simulink library "tqd"  (R2021b)
settings: Solver=VariableStepAuto  StartTime=0.0  StopTime=10.0  RelTol=1e-3
undefined symbols (not defined in the file or in its folder): ATQD_AccelLimitInRange_X_rpm, ATQD_AccelLimitInRange_Y_Nm, ATQD_AccelLimitOvrKi_X_Nm, ATQD_AccelLimitOvrKp_X_Nm, ATQD_BOSMapD_X_rpm, ATQD_BOSMapD_Y_pct, ATQD_BOSMapR_X_rpm, ATQD_BOSMapR_Y_pct, ATQD_HVBCurrSmooth_X_A, ATQD_LHMTqMapDLC_X_rpm, ATQD_LHMTqMapDLC_Y_pct, ATQD_LHMTqMapRLC_X_rpm, ATQD_LHMTqMapRLC_Y_pct, ATQD_NormalMapDLC_X_rpm, ATQD_NormalMapDLC_Y_pct, ATQD_NormalTqDecSR_X_rpm, ATQD_NormalTqDecSR_Y_Nm, ATQD_NormalTqIncSR_X_rpm, ATQD_NormalTqIncSR_Y_Nm, ATQD_OPDMapRLC_X_rpm, ATQD_OPDMapRLC_Y_pct, ATQD_RollRegTorReq_X_rpm, ATQD_RollRegTorReq_Y_enum, ATQD_VehSpdLimitInRange_X_rpm, ATQD_VehSpdLimitInRange_Y_Nm, ATQD_VehSpdLimitOvrKi_X_Nm, ATQD_VehSpdLimitOvrKp_X_Nm, EIGHT_INT, ENUM_BRAKEPEDAL_PRESSED, ENUM_BRAKEPEDAL_RELEASED, ENUM_COMBOKEY_DOWN, ENUM_COMBOKEY_M1, ENUM_COMBOKEY_M2, ENUM_COMBOKEY_NONE, ENUM_COMBOKEY_RKNEE, ENUM_COMBOKEY_STOPLV, ENUM_COMBOKEY_UP, ENUM_CP2VKNEEREQ_REQUEST, ENUM_CP2VNLVREQ_LEVEL1, ENUM_CP2VNLVREQ_LEVEL2, ENUM_CP2VNLVREQ_LOWER, ENUM_CP2VNLVREQ_STOPLV, ENUM_CP2VNLVREQ_UPPER, ENUM_CREEPIND_DISABLE, ENUM_CREEPIND_READY, ENUM_CREEPIND_RUNNING, ENUM_CREEPIND_WARNING, ENUM_DRIVELINERELEASE_RELEASE, ENUM_EBSTORQUERWQ_LIMIT, ENUM_EBSTORQUERWQ_TORQUE, ENUM_ECPVCUDRM_CONFORT, ENUM_ECPVCUDRM_ECO, ENUM_ECPVCUDRM_NORMAL, ENUM_ECPVCUDRM_NOTAVAILABLE, ENUM_EMTqModeDrvBrk_Accel, ENUM_EMTqModeDrvBrk_Brake, ENUM_EMTqModeDrvBrk_Coast, ENUM_ETC2ACTDRIVEDIR_BACKWARD, ENUM_ETC2ACTDRIVEDIR_FORWARD, ENUM_ETC2ACTDRIVEDIR_STILL ... (+341)
libraries: simulink x109, hcu_lib x67
(part 7 of 13)

== system tqd/TQD/Input_Convert/Function/Rolling Regen ==
  note: Torque Determination
  note: Enable Judgment
  BSCPIn_outputs : Inport
  BSignalConvert_outputs : Inport  Port=2
  VTQD_VCUMCUCtrlMdTQD_enum : Inport  Port=3
  AND : Logic  Inputs=8  AllPortsSameDT=off  OutDataTypeStr=boolean
  Bus Selector : BusSelector  OutputSignals=VTQD_EBSLostZeroReg_flg,VTQD_ActDriveMode_enum,VTQD_VCUVehSpd_kph
  Bus Selector1 : BusSelector  OutputSignals=VDHP_ActAPSPosn_pct,VINP_B2VAvaPlsChgCurr_A,VDMM_CAN1BUSOFF_flg,VINP_ECPVCURRegenSW_enum,VINP_EM1OvrCtrlMBrk_enum,VINP_MotorSpd_rpm,VINP_CANMsgValidECP3_flg
  Constant : Constant  Value=KTQD_RollRegAPSLimit_pct
  Constant1 : Constant  Value=KTQD_RollRegVehSpdLimit_kph
  Constant10 : Constant  Value=KTQD_RollingRegSW_enum_ovrdval
  Constant11 : Constant  Value=KTQD_RollingRegSW_enum_ovrdflg
  Constant12 : Constant  Value=KTQD_RollingRegSW_flg_ovrdflg
  Constant13 : Constant  Value=KTQD_RegenModeSW_flg
  Constant2 : Constant  Value=KTQD_RollRegBatAvalChgCurr_A
  Constant3 : Constant  Value=ENUM_MCUCTRLMODE_TORQUE
  Constant4 : Constant  Value=ZERO_FLOAT
  Constant5 : Constant  Value=KTQD_RollRegenIni_enum
  Constant6 : Constant  Value=KTQD_RollRegenThreshold_enum
  Constant7 : Constant  Value=ENUM_EBSTORQUERWQ_TORQUE
  Constant8 : Constant  Value=ZERO_INT
  Constant9 : Constant  Value=KTQD_RollingRegSW_flg_ovrdval
  Data Type Conversion : DataTypeConversion  OutDataTypeStr=single
  Data Type Conversion1 : DataTypeConversion  OutDataTypeStr=single
  Equal : RelationalOperator  Operator=~=  OutDataTypeStr=boolean  RndMeth=Simplest
  Gain1 : Gain  Gain=MINUSONE_FLOAT
  Gain2 : Gain  Gain=MINUSONE_FLOAT
  MTQD_RollRegTorReq_Z_Nm : Lookup_n-D  BreakpointsForDimension1=ATQD_RollRegTorReq_Y_enum  BreakpointsForDimension2=ATQD_RollRegTorReq_X_rpm  Table=MTQD_RollRegTorReq_Z_Nm  InternalRulePriority=Speed  RndMeth=Simplest  InputSameDT=on
      settings: InputPortMap=u0,u1
  MTQD_RollRegTorReq_Z_Nm1 : Lookup_n-D  BreakpointsForDimension1=ATQD_RollRegTorReq_Y_enum  BreakpointsForDimension2=ATQD_RollRegTorReq_X_rpm  Table=MTQD_RollRegTorReq_Z_Nm  InternalRulePriority=Speed  RndMeth=Simplest  InputSameDT=on
      settings: InputPortMap=u0,u1
  NOT : Logic  Operator=NOT  AllPortsSameDT=off  OutDataTypeStr=boolean
  NOT1 : Logic  Operator=NOT  AllPortsSameDT=off  OutDataTypeStr=boolean
  NOT2 : Logic  Operator=NOT  AllPortsSameDT=off  OutDataTypeStr=boolean
  OR : Logic  Operator=OR  AllPortsSameDT=off  OutDataTypeStr=boolean
  Relational Operator : RelationalOperator  Operator=<=  OutDataTypeStr=boolean  RndMeth=Simplest
  Relational Operator1 : RelationalOperator  OutDataTypeStr=boolean  RndMeth=Simplest
  Relational Operator2 : RelationalOperator  OutDataTypeStr=boolean  RndMeth=Simplest
  Relational Operator3 : RelationalOperator  Operator===  OutDataTypeStr=boolean  RndMeth=Simplest
  Relational Operator4 : RelationalOperator  Operator=>  OutDataTypeStr=boolean  RndMeth=Simplest
  Relational Operator5 : RelationalOperator  OutDataTypeStr=boolean  RndMeth=Simplest
  Switch{,2..4} (4 alike) : Switch  Criteria=u2 ~= 0
      settings: AttributesFormatString=%<Criteria>
  Switch1 : Switch  Criteria=u2 > Threshold
  VTQD_RollingRegenEnable_flg : Outport
  VTQD_RollRegTorReq_Nm : Outport  Port=2
  wires:
  [VTQD_RollingRegenEnable_flg] -> VTQD_RollingRegenEnable_flg/1
  BSCPIn_outputs/1 -> Bus Selector1/1
  Bus Selector/1 -> [VTQD_EBSLostZeroReg_flg]  "<VTQD_EBSLostZeroReg_flg>"
  BSignalConvert_outputs/1 -> Bus Selector/1
  [VINP_EM1OvrCtrlMBrk_enum] -> Equal/1
  Equal/1 -> AND/8
  Relational Operator5/1 -> Switch4/3
  Constant7/1 -> Equal/2
  Constant/1 -> Relational Operator/2
  Relational Operator2/1 -> AND/3
  Relational Operator1/1 -> AND/2
  [VDMM_CAN1BUSOFF_flg] -> NOT2/1
  [VINP_B2VAvaPlsChgCurr_A] -> Relational Operator2/1
  Relational Operator3/1 -> AND/4
  Relational Operator/1 -> AND/1
  [VTQD_VCUVehSpd_kph] -> Relational Operator1/1
  Constant8/1 -> Relational Operator5/2
  NOT1/1 -> AND/7
  Constant3/1 -> Relational Operator3/2
  Constant2/1 -> Relational Operator2/2
  [VINP_ECPVCURRegenSW_enum] -> Relational Operator5/1
  NOT2/1 -> AND/5
  Constant12/1 -> Switch4/2
  AND/1 -> [VTQD_RollingRegenEnable_flg]  "VTQD_RollingRegenEnable_flg"
  [VTQD_EBSLostZeroReg_flg] -> NOT1/1
  Switch4/1 -> AND/6
  Constant9/1 -> Switch4/1
  [VTQD_VCUMCUCtrlMdTQD_enum] -> Relational Operator3/1
  Constant1/1 -> Relational Operator1/2
  [VDHP_ActAPSPosn_pct] -> Relational Operator/1
  VTQD_VCUMCUCtrlMdTQD_enum/1 -> [VTQD_VCUMCUCtrlMdTQD_enum]
  MTQD_RollRegTorReq_Z_Nm1/1 -> Gain2/1
  Constant4/1 -> Switch/3
  Gain2/1 -> Switch1/3
  MTQD_RollRegTorReq_Z_Nm/1 -> Gain1/1
  Constant10/1 -> Switch3/1
  [VINP_MotorSpd_rpm] -> MTQD_RollRegTorReq_Z_Nm1/2
  Constant5/1 -> Data Type Conversion1/1
  Data Type Conversion1/1 -> MTQD_RollRegTorReq_Z_Nm/1
  [VINP_MotorSpd_rpm] -> MTQD_RollRegTorReq_Z_Nm/2
  Constant6/1 -> Relational Operator4/2
  Relational Operator4/1 -> OR/1
  [VINP_ECPVCURRegenSW_enum] -> Relational Operator4/1
  Switch3/1 -> Data Type Conversion/1
  OR/1 -> Switch1/2
  NOT/1 -> OR/2
  Gain1/1 -> Switch1/1
  Constant13/1 -> Switch2/2
  [VTQD_ActDriveMode_enum] -> Switch2/3
  Switch/1 -> [VTQD_RollRegTorReq_Nm]  "VTQD_RollRegTorReq_Nm"
  [VINP_CANMsgValidECP3_flg] -> NOT/1
  [VINP_ECPVCURRegenSW_enum] -> Switch2/1
  Switch1/1 -> Switch/1
  Constant11/1 -> Switch3/2
  [VTQD_RollingRegenEnable_flg] -> Switch/2
  Switch2/1 -> Switch3/3
  Data Type Conversion/1 -> MTQD_RollRegTorReq_Z_Nm1/1
  [VTQD_RollRegTorReq_Nm] -> VTQD_RollRegTorReq_Nm/1
  Bus Selector/2 -> [VTQD_ActDriveMode_enum]  "<VTQD_ActDriveMode_enum>"
  Bus Selector1/1 -> [VDHP_ActAPSPosn_pct]  "<VDHP_ActAPSPosn_pct>"
  Bus Selector1/2 -> [VINP_B2VAvaPlsChgCurr_A]  "<VINP_B2VAvaPlsChgCurr_A>"
  Bus Selector1/3 -> [VDMM_CAN1BUSOFF_flg]  "<VDMM_CAN1BUSOFF_flg>"
  Bus Selector1/4 -> [VINP_ECPVCURRegenSW_enum]  "<VINP_ECPVCURRegenSW_enum>"
  Bus Selector1/5 -> [VINP_EM1OvrCtrlMBrk_enum]  "<VINP_EM1OvrCtrlMBrk_enum>"
  Bus Selector1/6 -> [VINP_MotorSpd_rpm]  "<VINP_MotorSpd_rpm>"
  Bus Selector1/7 -> [VINP_CANMsgValidECP3_flg]  "<VINP_CANMsgValidECP3_flg>"
  Bus Selector/3 -> [VTQD_VCUVehSpd_kph]  "<VTQD_VCUVehSpd_kph>"

== system tqd/TQD/Input_Convert/Function/Shift Modul ==
  note: Actual Gear Position State Machine
  note: Shift Gear Command Judgment
  BSCPIn_outputs : Inport
  BSignalConvert_outputs : Inport  Port=2
  Bus Selector : BusSelector  OutputSignals=VTQD_DrivePositionOn_flg,VTQD_NeutralPositionOn_flg,VTQD_ReversePositionOn_flg,VTQD_BrkSWOn_flg,VTQD_EVDriveReady_flg,VTQD_IGNActive_flg,VTQD_EVCU1VehActDrvDir_enum,VTQD_GearFlashInd_flg,VTQD_DMSLossLimitGear_flg,VTQD_VCUVehSpd_kph
  Bus Selector1 : BusSelector  OutputSignals=task_time_s,VINP_MotorSpd_rpm,VDMM_DTCDMSRCIncorrect_flg,VINP_ParkBrakeSW_flg
  Constant : Constant  Value=ENUM_GEARSHIFTPOSN_R
  Constant1 : Constant  Value=ENUM_GEARSHIFTPOSN_INVALID
  Constant{10..14} (5 alike) : Constant  Value=FALSE
  Constant2 : Constant  Value=ENUM_GEARSHIFTPOSN_N
  Constant4 : Constant  Value=ENUM_GEARSHIFTPOSN_D
  Delay : Delay  DelayLength=1  InitialConditionSource=Input port
      settings: AttributesFormatString=%<InitialConditionSource>  InputPortMap=u0,p4
  Determine_Actual_Gear_Position : Stateflow chart  TreatAsAtomicUnit=on
  Logical Operator : Logic  Operator=OR  Inputs=3  AllPortsSameDT=off  OutDataTypeStr=boolean
  Switch1 : Switch  Criteria=u2 ~= 0
      settings: AttributesFormatString=%<Criteria>
  Switch3 : Switch  Criteria=u2 ~= 0
      settings: AttributesFormatString=%<Criteria>
  Switch4 : Switch  Criteria=u2 ~= 0
      settings: AttributesFormatString=%<Criteria>
  VTQD_GearActualPosn_enum : Outport
  VTQD_ParkingPawlPwrOn_flg : Outport  Port=2
  VTQD_ParkingPawlEnable_flg : Outport  Port=3
  wires:
  BSignalConvert_outputs/1 -> Bus Selector/1
  Delay/1 -> Switch3/3
  Constant/1 -> Switch3/1
  Constant2/1 -> Switch4/1
  Switch4/1 -> Delay/1, [VTQD_GearShiftPosn_enum]  "VTQD_GearShiftPosn_enum"
  Switch3/1 -> Switch1/3
  Logical Operator/1 -> [VTQD_RNDTrig_flg]  "VTQD_RNDTrig_flg"
  Constant4/1 -> Switch1/1
  Constant1/1 -> Delay/2
  Switch1/1 -> Switch4/3
  Bus Selector/1 -> [VTQD_DrivePositionOn_flg]  "<VTQD_DrivePositionOn_flg>"
  Bus Selector/2 -> [VTQD_NeutralPositionOn_flg]  "<VTQD_NeutralPositionOn_flg>"
  Bus Selector/3 -> [VTQD_ReversePositionOn_flg]  "<VTQD_ReversePositionOn_flg>"
  [VTQD_NeutralPositionOn_flg] -> Switch4/2
  [VTQD_DrivePositionOn_flg] -> Switch1/2
  [VTQD_ReversePositionOn_flg] -> Switch3/2
  [VTQD_ReversePositionOn_flg] -> Logical Operator/3
  [VTQD_DrivePositionOn_flg] -> Logical Operator/2
  [VTQD_NeutralPositionOn_flg] -> Logical Operator/1
  Determine_Actual_Gear_Position/3(VTQD_ParkingPawlEnable_flg) -> [VTQD_ParkingPawlEnable_flg]
  Determine_Actual_Gear_Position/2(VTQD_ParkingPawlPwrOn_flg) -> [VTQD_ParkingPawlPwrOn_flg]
  [VDMM_DTCDMSRCIncorrect_flg] -> Determine_Actual_Gear_Position/17(VDMM_DTCDMSRCIncorrect_flg)
  [VINP_ParkBrakeSW_flg] -> Determine_Actual_Gear_Position/18(VINP_ParkBrakeSW_flg)
  [VTQD_GearFlashInd_flg] -> Determine_Actual_Gear_Position/14(VSCP_GearFlashInd_flg)
  [VTQD_EVCU1VehActDrvDir_enum] -> Determine_Actual_Gear_Position/13(VSCP_EVCU1VehActDrvDir_enum)
  [VTQD_EVDriveReady_flg] -> Determine_Actual_Gear_Position/6(VFUN_EVDriveReady_flg)
  [VTQD_tasktime_s] -> Determine_Actual_Gear_Position/5(task_time_s)
  [VTQD_BrkSWOn_flg] -> Determine_Actual_Gear_Position/4(VINP_BrkSwOn_flg)
  [VINP_MotorSpd_rpm] -> Determine_Actual_Gear_Position/16(VINP_TMSpd_rpm)
  [VTQD_DMSLossLimitGear_flg] -> Determine_Actual_Gear_Position/15(VTQD_DMSLossLimitGear_flg)
  [VTQD_GearShiftPosn_enum] -> Determine_Actual_Gear_Position/1(VTQD_GearShiftPosn_enum)
  [VTQD_VCUVehSpd_kph] -> Determine_Actual_Gear_Position/2(VINP_VehSpd_kph)
  [VTQD_RNDTrig_flg] -> Determine_Actual_Gear_Position/8(VTQD_RNDTrig_flg)
  Constant12/1 -> Determine_Actual_Gear_Position/10(VTQD_ADASModeDisact_flg)  "VTQD_ADASModeDisact_flg"
  [VTQD_IGNActive_flg] -> Determine_Actual_Gear_Position/7(VPSA_IGNActive_flg)
  Determine_Actual_Gear_Position/1(VTQD_GearActualPosn_enum) -> [VTQD_GearActualPosn_enum]
  BSCPIn_outputs/1 -> Bus Selector1/1
  Constant10/1 -> Determine_Actual_Gear_Position/3(VINP_ParkingPawlLock_flg)  "VINP_ParkingPawlLock_flg"
  Bus Selector/4 -> [VTQD_BrkSWOn_flg]  "<VTQD_BrkSWOn_flg>"
  Bus Selector/5 -> [VTQD_EVDriveReady_flg]  "<VTQD_EVDriveReady_flg>"
  Bus Selector/6 -> [VTQD_IGNActive_flg]  "<VTQD_IGNActive_flg>"
  Constant11/1 -> Determine_Actual_Gear_Position/9(VTQD_AutoPark_flg)  "VTQD_AutoPark_flg"
  Constant13/1 -> Determine_Actual_Gear_Position/11(VTQD_ExtShiftAvail_flg)  "VTQD_ExtShiftAvail_flg"
  Constant14/1 -> Determine_Actual_Gear_Position/12(VINP_ADASShftPosnReqA_flg)  "VINP_ADASShftPosnReqA_flg"
  Bus Selector/7 -> [VTQD_EVCU1VehActDrvDir_enum]  "<VTQD_EVCU1VehActDrvDir_enum>"
  Bus Selector/8 -> [VTQD_GearFlashInd_flg]  "<VTQD_GearFlashInd_flg>"
  Bus Selector/9 -> [VTQD_DMSLossLimitGear_flg]  "<VTQD_DMSLossLimitGear_flg>"
  [VTQD_GearActualPosn_enum] -> VTQD_GearActualPosn_enum/1
  [VTQD_ParkingPawlPwrOn_flg] -> VTQD_ParkingPawlPwrOn_flg/1
  [VTQD_ParkingPawlEnable_flg] -> VTQD_ParkingPawlEnable_flg/1
  Bus Selector1/1 -> [VTQD_tasktime_s]  "<task_time_s>"
  Bus Selector1/2 -> [VINP_MotorSpd_rpm]  "<VINP_MotorSpd_rpm>"
  Bus Selector1/3 -> [VDMM_DTCDMSRCIncorrect_flg]  "<VDMM_DTCDMSRCIncorrect_flg>"
  Bus Selector1/4 -> [VINP_ParkBrakeSW_flg]  "<VINP_ParkBrakeSW_flg>"
  Bus Selector/10 -> [VTQD_VCUVehSpd_kph]  "<VTQD_VCUVehSpd_kph>"

== system tqd/TQD/Input_Convert/Function/Speed Limiter ==
  note: Limit Speed Determination
  note: Torque Calculation
  note: Enable Judgment
  note: Signal Convert
  BSCPIn_outputs : Inport
  BSignalConvert_outputs : Inport  Port=2
  VTQD_GearActualPosn_enum : Inport  Port=3
  VTQD_PedalMapTq_Nm : Inport  Port=4
  AND : Logic  Inputs=6  AllPortsSameDT=off  OutDataTypeStr=boolean
  Add2 : Sum  Inputs=+-
  Add4 : Sum
  Bus Selector : BusSelector  OutputSignals=VTQD_PTAvailMotTq_Nm,VTQD_VCUVehSpd_kph
  Bus Selector1 : BusSelector  OutputSignals=task_time_s,VINP_ECPVCUSpdLim_kph,VINP_CANMsgValidECP2_flg,VINP_FASpeedValid_flg,VINP_MotorSpdValid_flg,VINP_ECPVCUSpdLimSw_flg,VINP_MotorSpd_rpm
  Constant : Constant  Value=SINGLEMAXCNT  OutDataTypeStr=single
  Constant1 : Constant  Value=KTQD_VehSpdLimitTG_kph
  Constant10 : Constant  Value=KTQD_VehSpdLimitSW_flg_ovrdval
  Constant11 : Constant  Value=KTQD_VehSpdOvrLimitRefreTime_s
  Constant12 : Constant  Value=KTQD_VehSpdLimitOvrRangeDis_kph
  Constant14 : Constant  Value=KTQD_VehSpdLimitTorLowerLim_Nm
  Constant15 : Constant  Value=KTQD_MCUMaxRefTorq_Nm
  Constant16 : Constant  Value=KTQD_VehSpdLimitSW_flg_ovrdflg
  Constant2 : Constant  Value=KTQD_VehSpdPhyShrehold_kph
  Constant3 : Constant  Value=KTQD_VehSpdLimitExtre_kph
  Constant4 : Constant  Value=KTQD_ECPSetValErr1_kph
  Constant5 : Constant  Value=KTQD_VehSpdLimitTG_kph
  Constant6 : Constant  Value=KTQD_ECPSetValNoReq_kph
  Constant7 : Constant  Value=ENUM_GEARACTUALPOSN_D
  Constant8 : Constant  Value=KTQD_VehSpdLimitInRangeDis_kph
  Constant9 : Constant  Value=KTQD_VehSpdOvrLimitRefreTime_s
  Counter : hcu_lib/Basic_Blocks/Counter
  Data Type Conversion : DataTypeConversion  OutDataTypeStr=single
  Detect Increase1 : simulink/Logic and Bit Operations/Detect Increase  vinit=boolean(0)  OutDataTypeStr=boolean
  Detect Increase3 : simulink/Logic and Bit Operations/Detect Increase  vinit=boolean(0)  OutDataTypeStr=boolean
  Equal : RelationalOperator  Operator===  OutDataTypeStr=boolean  RndMeth=Simplest
  Limit Torque Calculation : Subsystem  TreatAsAtomicUnit=on
  Limit2 : hcu_lib/Basic_Blocks/Limit
  MTQD_VehSpdLimitInRange_Z_Gain : Lookup_n-D  BreakpointsForDimension1=ATQD_VehSpdLimitInRange_Y_Nm  BreakpointsForDimension2=ATQD_VehSpdLimitInRange_X_rpm  Table=MTQD_VehSpdLimitInRange_Z_Gain  InternalRulePriority=Speed  RndMeth=Simplest  InputSameDT=on
      settings: InputPortMap=u0,u1
  Min : MinMax  Inputs=2
  NOT : Logic  Operator=NOT  AllPortsSameDT=off  OutDataTypeStr=boolean
  NOT1 : Logic  Operator=NOT  AllPortsSameDT=off  OutDataTypeStr=boolean
  NOT2 : Logic  Operator=NOT  AllPortsSameDT=off  OutDataTypeStr=boolean
  OR : Logic  Operator=OR  AllPortsSameDT=off  OutDataTypeStr=boolean
  Product : Product
  Product1 : Product
  Relational Operator{1..4} (4 alike) : RelationalOperator  OutDataTypeStr=boolean  RndMeth=Simplest
  Relational Operator11 : RelationalOperator  Operator=<  OutDataTypeStr=boolean  RndMeth=Simplest
  Relational Operator9 : RelationalOperator  Operator=<=  OutDataTypeStr=boolean  RndMeth=Simplest
  SR_Latch : hcu_lib/Basic_Blocks/SR_Latch
  Saturation : Saturate  UpperLimit=KTQD_MCUMaxRefTorq_Nm  LowerLimit=ZERO_FLOAT
      settings: AttributesFormatString=|
      | UpperLimit:%<UpperLimit>
      | LowerLimit:%<LowerLimit>
  Saturation1 : Saturate  UpperLimit=KTQD_EMSpdAcclLimitEnHi_rpm  LowerLimit=ZERO_FLOAT
      settings: AttributesFormatString=|
      | UpperLimit:%<UpperLimit>
      | LowerLimit:%<LowerLimit>
  Switch{1..3,5,10,12..13} (7 alike) : Switch  Criteria=u2 ~= 0
      settings: AttributesFormatString=%<Criteria>
  Unit Delay : UnitDelay  InitialCondition=boolean(0)  SampleTime=-1  HasFrameUpgradeWarning=on
      settings: AttributesFormatString=%<InitialCondition>
  Unit Delay1 : UnitDelay  InitialCondition=single(0)  SampleTime=-1  HasFrameUpgradeWarning=on
      settings: AttributesFormatString=%<InitialCondition>
  Unit Delay12 : UnitDelay  InitialCondition=THOUSAND  SampleTime=-1  HasFrameUpgradeWarning=on
      settings: AttributesFormatString=%<InitialCondition>
  VTQD_VehSpdLimitEnable_flg : Outport
  VTQD_VehSpdLimitTG_kph : Outport  Port=2
  VTQD_VehSpdTorLimit_Nm : Outport  Port=3
  wires:
  [VTQD_VehSpdLimitEnable_flg] -> VTQD_VehSpdLimitEnable_flg/1
  BSCPIn_outputs/1 -> Bus Selector1/1
  Bus Selector/1 -> [VTQD_PTAvailMotTq_Nm]  "<VTQD_PTAvailMotTq_Nm>"
  BSignalConvert_outputs/1 -> Bus Selector/1
  Constant2/1 -> Switch2/3
  [VTQD_VehSpdLimitEnable_flg] -> Switch2/2
  Switch2/1 -> [VTQD_VehSpdLimitRef_kph]  "VTQD_VehSpdLimitRef_kph"
  [VTQD_VehSpdLimitTG_kph] -> Switch2/1
  [VTQD_VehSpdLimitRef_kph] -> Add2/1
  Add2/1 -> Relational Operator1/2
  Add4/1 -> Relational Operator3/2
  Relational Operator1/1 -> [VTQD_VehSpdInLimit_flg]  "VTQD_VehSpdInLimit_flg"
  [VTQD_VCUVehSpd_kph] -> Relational Operator3/1
  Constant8/1 -> Add2/2
  [VTQD_VCUVehSpd_kph] -> Relational Operator1/1
  [VTQD_VehSpdLimitRef_kph] -> Add4/1
  Relational Operator4/1 -> [VTQD_VehSpdOvrRef_flg]  "VTQD_VehSpdOvrRef_flg"
  [VTQD_VehSpdLimitRef_kph] -> Relational Operator4/2
  Constant12/1 -> Add4/2
  [VTQD_VCUVehSpd_kph] -> Relational Operator4/1
  Relational Operator3/1 -> [VTQD_VehSpdOvrLimit_flg]  "VTQD_VehSpdOvrLimit_flg"
  [task_time_s] -> Product/2
  Product/1 -> Relational Operator2/1
  [VTQD_VehSpdOvrLimit_flg] -> NOT1/1, Counter/1
  Constant/1 -> Counter/3
  Unit Delay/1 -> OR/2
  Counter/1 -> Product/1
  OR/1 -> Counter/2
  Constant9/1 -> Relational Operator2/2
  Relational Operator2/1 -> [VTQD_VehSpdContiOvrLimit_flg], Unit Delay/1  "VTQD_VehSpdContiOvrLimit_flg"
  NOT1/1 -> OR/1
  [VINP_FASpeedValid_flg] -> AND/3
  AND/1 -> [VTQD_VehSpdLimitEnable_flg]  "VTQD_VehSpdLimitEnable_flg"
  [VINP_MotorSpdValid_flg] -> AND/5
  Constant4/1 -> Relational Operator11/2
  Switch5/1 -> AND/6
  Constant7/1 -> Equal/2
  [VINP_ECPVCUSpdLim_kph] -> Relational Operator11/1
  Equal/1 -> AND/1
  Relational Operator11/1 -> AND/4
  [VINP_CANMsgValidECP2_flg] -> AND/2
  [VTQD_GearActualPosn_enum] -> Equal/1
  Constant16/1 -> Switch5/2
  Constant10/1 -> Switch5/1
  [VINP_ECPVCUSpdLimSw_flg] -> Switch5/3
  [VINP_MotorSpd_rpm] -> Saturation1/1
  SR_Latch/1 -> NOT2/1
  Data Type Conversion/1 -> Switch12/1
  NOT/1 -> SR_Latch/2
  Switch13/1 -> Switch10/3
  Switch12/1 -> Limit2/1
  Constant15/1 -> Limit2/2
  [VTQD_VCUVehSpd_kph] -> Limit Torque Calculation/2(VDIP_VCUVehSpd_kph)
  [VTQD_VehSpdContiOvrLimit_flg] -> Limit Torque Calculation/Trigger
  Limit2/1 -> [VTQD_VehSpdTorLimit_Nm]  "VTQD_VehSpdTorLimit_Nm"
  Detect Increase1/1 -> SR_Latch/1
  Saturation/1 -> MTQD_VehSpdLimitInRange_Z_Gain/1
  [VTQD_PedalMapTq_Nm] -> Product1/2
  Saturation1/1 -> MTQD_VehSpdLimitInRange_Z_Gain/2
  MTQD_VehSpdLimitInRange_Z_Gain/1 -> Product1/1
  [VTQD_VehSpdInLimit_flg] -> Detect Increase1/1
  [VTQD_VehSpdContiOvrLimit_flg] -> Switch12/2
  [VTQD_PTAvailMotTq_Nm] -> Switch13/1
  Detect Increase3/1 -> Switch10/2
  Switch10/1 -> Switch12/3
  Unit Delay12/1 -> Switch13/3
  [VTQD_VehSpdInLimit_flg] -> Detect Increase3/1
  [VTQD_VehSpdOvrRef_flg] -> NOT/1
  [VTQD_VehSpdTorLimit_Nm] -> Unit Delay12/1
  Limit Torque Calculation/1(Result) -> Data Type Conversion/1
  [VTQD_VehSpdTorLimit_Nm] -> Unit Delay1/1
  [VTQD_PedalMapTq_Nm] -> Saturation/1
  Product1/1 -> Switch10/1
  Constant11/1 -> Limit Torque Calculation/3(PIControl_Task_time)
  Unit Delay1/1 -> Limit Torque Calculation/4(VTQD_VehSpdTorLimitLast_Nm)
  Constant14/1 -> Limit2/3
  [VTQD_VehSpdLimitRef_kph] -> Limit Torque Calculation/1(Refference)
  NOT2/1 -> Switch13/2
  Min/1 -> Switch3/1
  [VTQD_VehSpdLimitEnable_flg] -> Switch3/2
  Constant3/1 -> Switch3/3
  Switch1/1 -> Min/2
  Constant5/1 -> Switch1/1
  [VINP_ECPVCUSpdLim_kph] -> Relational Operator9/1
  Constant1/1 -> Min/1
  Relational Operator9/1 -> Switch1/2
  [VINP_ECPVCUSpdLim_kph] -> Switch1/3
  Constant6/1 -> Relational Operator9/2
  Switch3/1 -> [VTQD_VehSpdLimitTG_kph]  "VTQD_VehSpdLimitTG_kph"
  VTQD_GearActualPosn_enum/1 -> [VTQD_GearActualPosn_enum]
  VTQD_PedalMapTq_Nm/1 -> [VTQD_PedalMapTq_Nm]
  [VTQD_VehSpdLimitTG_kph] -> VTQD_VehSpdLimitTG_kph/1
  [VTQD_VehSpdTorLimit_Nm] -> VTQD_VehSpdTorLimit_Nm/1
  Bus Selector/2 -> [VTQD_VCUVehSpd_kph]  "<VTQD_VCUVehSpd_kph>"
  Bus Selector1/1 -> [task_time_s]  "<task_time_s>"
  Bus Selector1/2 -> [VINP_ECPVCUSpdLim_kph]  "<VINP_ECPVCUSpdLim_kph>"
  Bus Selector1/3 -> [VINP_CANMsgValidECP2_flg]  "<VINP_CANMsgValidECP2_flg>"
  Bus Selector1/4 -> [VINP_FASpeedValid_flg]  "<VINP_FASpeedValid_flg>"
  Bus Selector1/5 -> [VINP_MotorSpdValid_flg]  "<VINP_MotorSpdValid_flg>"
  Bus Selector1/6 -> [VINP_ECPVCUSpdLimSw_flg]  "<VINP_ECPVCUSpdLimSw_flg>"
  Bus Selector1/7 -> [VINP_MotorSpd_rpm]  "<VINP_MotorSpd_rpm>"

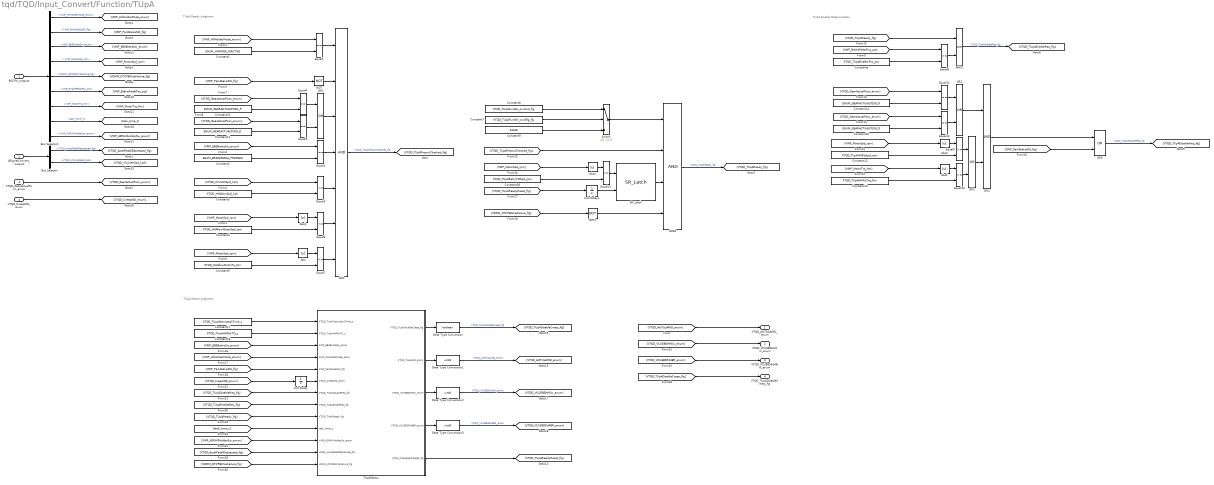
== system tqd/TQD/Input_Convert/Function/TUpA ==
  note: TUpA Status Judgment
  note: TUpA Ready Judgment
  note: TUpA Enable Determination
  BSCPIn_outputs : Inport
  BSignalConvert_outputs : Inport  Port=2
  VTQD_GearActualPosn_enum : Inport  Port=3
  VTQD_CreepIND_enum : Inport  Port=4
  AND : Logic  Inputs=7  AllPortsSameDT=off  OutDataTypeStr=boolean
  AND1 : Logic  AllPortsSameDT=off  OutDataTypeStr=boolean
  AND2 : Logic  Inputs=4  AllPortsSameDT=off  OutDataTypeStr=boolean
  Abs{,1..4} (5 alike) : Abs
  Bus Selector : BusSelector  OutputSignals=VTQD_AccelPedalDepressed_flg,VTQD_VCUVehSpd_kph
  Bus Selector1 : BusSelector  OutputSignals=VINP_HillHolderMode_enum,VINP_ParkBrakeSW_flg,VINP_EBSBrakeSw_enum,VINP_MotorSpd_rpm,VDMM_DTCPBWireFailure_flg,VINP_BrakePedalPos_pct,VINP_MotorTrq_Nm,task_time_s,VINP_ASRHillHolderSw_enum
  Constant1 : Constant  Value=ENUM_HHMODE_INACTIVE
  Constant10 : Constant  Value=ENUM_GEARACTUALPOSN_R
  Constant11 : Constant  Value=ENUM_GEARACTUALPOSN_D
  Constant12 : Constant  Value=KTQD_TUpAHHRlsSpd_rpm
  Constant13 : Constant  Value=KTQD_TUpAHHRlsTrq_Nm
  Constant14 : Constant  Value=ENUM_GEARACTUALPOSN_R
  Constant15 : Constant  Value=ENUM_GEARACTUALPOSN_D
  Constant16 : Constant  Value=KTQD_TUpAHHFbkTO_s
  Constant17 : Constant  Value=KTQD_TUpAWarnLatchTime_s
  Constant18 : Constant  Value=KTQD_TUpARetryTMSpd_rpm
  Constant2 : Constant  Value=ENUM_BRAKEPEDAL_PRESSED
  Constant3 : Constant  Value=KTQD_HHAllowSpd_kph
  Constant4 : Constant  Value=KTQD_HHAllowMotorSpd_rpm
  Constant5 : Constant  Value=KTQD_HHAllowMotorTq_Nm
  Constant6 : Constant  Value=KTQD_TUpAEnaBrkPos_pct
  Constant7 : Constant  Value=KTQD_TUpAFuncEn_ovrdflg_flg
  Constant8 : Constant  Value=KTQD_TUpAFuncEn_ovrdval_flg
  Constant9 : Constant  Value=FALSE
  Data Type Conversion : DataTypeConversion  OutDataTypeStr=boolean
  Data Type Conversion1 : DataTypeConversion  OutDataTypeStr=uint8
  Data Type Conversion2 : DataTypeConversion  OutDataTypeStr=uint8
  Data Type Conversion3 : DataTypeConversion  OutDataTypeStr=uint8
  Equal{1..2,4..5,11..12} (6 alike) : RelationalOperator  Operator===  OutDataTypeStr=boolean  RndMeth=Simplest
  Equal{8..10,13} (4 alike) : RelationalOperator  OutDataTypeStr=boolean  RndMeth=Simplest
  Equal3 : RelationalOperator  Operator=<=  OutDataTypeStr=boolean  RndMeth=Simplest
  Equal6 : RelationalOperator  Operator=<=  OutDataTypeStr=boolean  RndMeth=Simplest
  Equal7 : RelationalOperator  Operator=<=  OutDataTypeStr=boolean  RndMeth=Simplest
  NOT : Logic  Operator=NOT  AllPortsSameDT=off  OutDataTypeStr=boolean
  NOT1 : Logic  Operator=NOT  AllPortsSameDT=off  OutDataTypeStr=boolean
  OR{1..3,5} (4 alike) : Logic  Operator=OR  AllPortsSameDT=off  OutDataTypeStr=boolean
  OR4 : Logic  AllPortsSameDT=off  OutDataTypeStr=boolean
  SR_Latch : hcu_lib/Basic_Blocks/SR_Latch
      settings: SourceProductName=HCU Relative Block Library
  Switch : Switch  Criteria=u2 ~= 0
      settings: AttributesFormatString=%<Criteria>
  TUpAStatus : Stateflow chart  AncestorBlock=tqd_T1_A08133TT4/TQD/TorqueDemand/TorqueModule/TUpA/TUpAStatus  TreatAsAtomicUnit=on
  Unit Delay : UnitDelay  InitialCondition=uint8(0)  SampleTime=-1  HasFrameUpgradeWarning=on
      settings: AttributesFormatString=%<InitialCondition>
  Unit Delay1 : UnitDelay  InitialCondition=boolean(0)  SampleTime=-1  HasFrameUpgradeWarning=on
      settings: AttributesFormatString=%<InitialCondition>
  VTQD_ActTUpAIND_enum : Outport
  VTQD_VCUEBSHHSw_enum : Outport  Port=2
  VTQD_VCUEBSRd4BR_enum : Outport  Port=3
  VTQD_TUpADisableCreep_flg : Outport  Port=4
  wires:
  [VTQD_ActTUpAIND_enum] -> VTQD_ActTUpAIND_enum/1
  BSCPIn_outputs/1 -> Bus Selector1/1
  Bus Selector/1 -> [VTQD_AccelPedalDepressed_flg]  "<VTQD_AccelPedalDepressed_flg>"
  BSignalConvert_outputs/1 -> Bus Selector/1
  [VTQD_TUpAPreconChecked_flg] -> AND2/2
  Switch/1 -> AND2/1
  Constant2/1 -> Equal2/2
  Equal6/1 -> AND/6
  AND/1 -> [VTQD_TUpAPreconChecked_flg]  "VTQD_TUpAPreconChecked_flg"
  [VINP_EBSBrakeSw_enum] -> Equal2/1
  [VINP_ParkBrakeSW_flg] -> NOT/1
  [VTQD_VCUVehSpd_kph] -> Equal3/1
  Equal4/1 -> OR1/1
  Constant10/1 -> Equal4/2
  NOT1/1 -> AND2/4
  Constant5/1 -> Equal7/2
  Constant3/1 -> Equal3/2
  Constant4/1 -> Equal6/2
  [VTQD_TUpAReadyReset_flg] -> Unit Delay1/1
  Equal7/1 -> AND/7
  Constant1/1 -> Equal1/2
  [VINP_HillHolderMode_enum] -> Equal1/1
  Equal1/1 -> AND/1
  Constant9/1 -> Switch/3
  OR1/1 -> AND/3
  [VINP_MotorSpd_rpm] -> Abs3/1
  [VTQD_GearActualPosn_enum] -> Equal4/1
  Constant7/1 -> Switch/2
  [VINP_MotorSpd_rpm] -> Abs4/1
  Equal13/1 -> SR_Latch/1
  Abs4/1 -> Equal13/1
  Abs3/1 -> Equal6/1
  Equal5/1 -> OR1/2
  Constant18/1 -> Equal13/2
  Abs/1 -> Equal7/1
  [VDMM_DTCPBWireFailure_flg] -> NOT1/1
  Equal2/1 -> AND/4
  Constant8/1 -> Switch/1
  [VINP_MotorSpd_rpm] -> Abs/1
  Unit Delay1/1 -> SR_Latch/2
  SR_Latch/1 -> AND2/3
  AND2/1 -> [VTQD_TUpAReady_flg]  "VTQD_TUpAReady_flg"
  [VTQD_GearActualPosn_enum] -> Equal5/1
  Equal3/1 -> AND/5
  Constant11/1 -> Equal5/2
  NOT/1 -> AND/2
  VTQD_GearActualPosn_enum/1 -> [VTQD_GearActualPosn_enum]
  OR5/1 -> [VTQD_TUpADisableReq_flg]  "VTQD_TUpADisableReq_flg"
  Equal9/1 -> OR3/1
  Constant12/1 -> Equal9/2
  [VINP_MotorTrq_Nm] -> Abs1/1
  Abs2/1 -> Equal9/1
  Equal8/1 -> AND1/2
  AND1/1 -> [VTQD_TUpAEnableReq_flg]  "VTQD_TUpAEnableReq_flg"
  [VINP_MotorSpd_rpm] -> Abs2/1
  OR2/1 -> OR4/1
  [VTQD_GearActualPosn_enum] -> Equal11/1
  Constant13/1 -> Equal10/2
  OR3/1 -> OR4/2
  Equal10/1 -> OR3/2
  [VTQD_GearActualPosn_enum] -> Equal12/1
  Equal12/1 -> OR2/2
  [VINP_ParkBrakeSW_flg] -> OR5/2
  [VINP_BrakePedalPos_pct] -> Equal8/1
  [VTQD_TUpAReady_flg] -> AND1/1
  Abs1/1 -> Equal10/1
  Equal11/1 -> OR2/1
  Constant15/1 -> Equal12/2
  Constant6/1 -> Equal8/2
  OR4/1 -> OR5/1
  Constant14/1 -> Equal11/2
  Unit Delay/1 -> TUpAStatus/6(VTQD_CreepIND_enum)
  Data Type Conversion/1 -> [VTQD_TUpADisableCreep_flg]  "VTQD_TUpADisableCreep_flg"
  [VTQD_CreepIND_enum] -> Unit Delay/1
  Data Type Conversion3/1 -> [VTQD_VCUEBSRd4BR_enum]  "VTQD_VCUEBSRd4BR_enum"
  [VTQD_TUpADisableReq_flg] -> TUpAStatus/7(VTQD_TUpADisableReq_flg)
  TUpAStatus/4(VTQD_VCUEBSRd4BR_enum) -> Data Type Conversion3/1
  [VINP_ParkBrakeSW_flg] -> TUpAStatus/5(VINP_ParkBreakSW_flg)
  [VTQD_TUpAReady_flg] -> TUpAStatus/9(VTQD_TUpAReady_flg)
  Constant16/1 -> TUpAStatus/2(KTQD_TUpAHHFbkTO_s)
  [VINP_ASRHillHolderSw_enum] -> TUpAStatus/11(VINP_ASRHillHolderSw_enum)
  TUpAStatus/1(VTQD_TUpADisableCreep_flg) -> Data Type Conversion/1
  Data Type Conversion1/1 -> [VTQD_ActTUpAIND_enum]  "VTQD_ActTUpAIND_enum"
  [task_time_s] -> TUpAStatus/10(task_time_s)
  Constant17/1 -> TUpAStatus/1(KTQD_TUpAWarnLatchTime_s)
  TUpAStatus/3(VTQD_VCUEBSHHSw_enum) -> Data Type Conversion2/1
  TUpAStatus/2(VTQD_TUpAIND_enum) -> Data Type Conversion1/1
  Data Type Conversion2/1 -> [VTQD_VCUEBSHHSw_enum]  "VTQD_VCUEBSHHSw_enum"
  [VINP_EBSBrakeSw_enum] -> TUpAStatus/3(VINP_EBSBrakeSw_enum)
  [VINP_HillHolderMode_enum] -> TUpAStatus/4(VINP_HillHolderMode_enum)
  [VTQD_TUpAEnableReq_flg] -> TUpAStatus/8(VTQD_TUpAEnableReq_flg)
  TUpAStatus/5(VTQD_TUpAReadyReset_flg) -> [VTQD_TUpAReadyReset_flg]
  [VDMM_DTCPBWireFailure_flg] -> TUpAStatus/13(VDMM_DTCPBWireFailure_flg)
  [VTQD_AccelPedalDepressed_flg] -> TUpAStatus/12(VDHP_AccelPedalDepressed_flg)
  VTQD_CreepIND_enum/1 -> [VTQD_CreepIND_enum]
  [VTQD_VCUEBSHHSw_enum] -> VTQD_VCUEBSHHSw_enum/1
  [VTQD_VCUEBSRd4BR_enum] -> VTQD_VCUEBSRd4BR_enum/1
  [VTQD_TUpADisableCreep_flg] -> VTQD_TUpADisableCreep_flg/1
  Bus Selector/2 -> [VTQD_VCUVehSpd_kph]  "<VTQD_VCUVehSpd_kph>"
  Bus Selector1/1 -> [VINP_HillHolderMode_enum]  "<VINP_HillHolderMode_enum>"
  Bus Selector1/2 -> [VINP_ParkBrakeSW_flg]  "<VINP_ParkBrakeSW_flg>"
  Bus Selector1/3 -> [VINP_EBSBrakeSw_enum]  "<VINP_EBSBrakeSw_enum>"
  Bus Selector1/4 -> [VINP_MotorSpd_rpm]  "<VINP_MotorSpd_rpm>"
  Bus Selector1/5 -> [VDMM_DTCPBWireFailure_flg]  "<VDMM_DTCPBWireFailure_flg>"
  Bus Selector1/6 -> [VINP_BrakePedalPos_pct]  "<VINP_BrakePedalPos_pct>"
  Bus Selector1/7 -> [VINP_MotorTrq_Nm]  "<VINP_MotorTrq_Nm>"
  Bus Selector1/8 -> [task_time_s]  "<task_time_s>"
  Bus Selector1/9 -> [VINP_ASRHillHolderSw_enum]  "<VINP_ASRHillHolderSw_enum>"

== system tqd/TQD/Input_Convert/Function/Torque Capacity ==
  note: Generating Torque Capacity
  note: Motoring Torque Capacity
  BSCPIn_outputs : Inport
  BSignalConvert_outputs : Inport  Port=2
  Abs : Abs
  Abs1 : Abs
  Bus Selector1 : BusSelector  OutputSignals=task_time_s,VINP_B2VAvaPlsChgCurr_A,VINP_MotorSpd_rpm,VINP_B2VAPlsDischgCurr_A,VINP_B2VPackInsideVol_V,VINP_B2VPackCurr_A,VINP_HVBPwrAvailDchrgValid_flg,VINP_B2VAvaPlsChgCurrValid_flg,VINP_MCUTrqLimHi_Nm,VINP_MCUTrqLimLo_Nm
  Constant1 : Constant  Value=THOUSAND
  Constant2 : Constant  Value=KTQD_HVBattAvailPwrDefMot_Nm
  Constant3 : Constant  Value=EPS
  Constant4 : Constant  Value=THOUSAND
  Constant5 : Constant  Value=EPS
  Constant6 : Constant  Value=KTQD_HVBattAvailPwrDefGen_Nm
  Data Type Conversion : DataTypeConversion  OutDataTypeStr=single
  Data Type Conversion1 : DataTypeConversion  OutDataTypeStr=single
  Divide : Product  Inputs=**/
  Divide1 : Product  Inputs=**/
  Fcn : Fcn  Expr=u[1]/u[2]/pi*30000
  Fcn1 : Fcn  Expr=u[1]/u[2]/pi*30000
  FirstOrderFilter8 : hcu_lib/Basic_Blocks/FirstOrderFilter
      settings: SourceProductName=HCU Relative Block Library
  Gain : Gain  Gain=MINUSONE_FLOAT
  MTQD_HVBCurrSmooth_Y_gain : Lookup_n-D  NumberOfTableDimensions=1  BreakpointsForDimension1=ATQD_HVBCurrSmooth_X_A  Table=MTQD_HVBCurrSmooth_Y_gain  InternalRulePriority=Speed  RndMeth=Simplest  InputSameDT=on
  Max : MinMax  Function=max  Inputs=2
  Max1 : MinMax  Function=max  Inputs=2
  Min : MinMax  Inputs=2
  Min1 : MinMax  Function=max  Inputs=2
  Mux : Mux  Inputs=2
  Mux1 : Mux  Inputs=2
  Saturaton : Saturate  UpperLimit=5000  LowerLimit=100
      settings: AttributesFormatString=|
      | UpperLimit:%<UpperLimit>
      | LowerLimit:%<LowerLimit>
  Saturaton1 : Saturate  UpperLimit=3000  LowerLimit=0
      settings: AttributesFormatString=|
      | UpperLimit:%<UpperLimit>
      | LowerLimit:%<LowerLimit>
  Saturaton2 : Saturate  UpperLimit=5000  LowerLimit=100
      settings: AttributesFormatString=|
      | UpperLimit:%<UpperLimit>
      | LowerLimit:%<LowerLimit>
  Saturaton3 : Saturate  UpperLimit=3000  LowerLimit=0
      settings: AttributesFormatString=|
      | UpperLimit:%<UpperLimit>
      | LowerLimit:%<LowerLimit>
  Switch : Switch  Criteria=u2 ~= 0
      settings: AttributesFormatString=%<Criteria>
  Switch1 : Switch  Criteria=u2 ~= 0
      settings: AttributesFormatString=%<Criteria>
  Terminator : Terminator
  VTQD_TMTqCapMot_Nm : Outport
  VTQD_TMTqCapGen_Nm : Outport  Port=2
  wires:
  [VINP_MotorSpd_rpm] -> Abs/1
  Abs/1 -> Saturaton/1
  [VTQD_HVBPwrAvailDchrg_kW] -> Mux/1
  Saturaton/1 -> Mux/2
  Mux/1 -> Fcn/1
  Fcn/1 -> Saturaton1/1
  Saturaton1/1 -> [VTQD_HVBDischrgLim_Nm]  "VTQD_HVBDischrgLim_Nm"
  [VTQD_HVBDischrgLim_Nm] -> FirstOrderFilter8/1
  [task_time_s] -> FirstOrderFilter8/2
  [VINP_B2VPackCurr_A] -> MTQD_HVBCurrSmooth_Y_gain/1
  MTQD_HVBCurrSmooth_Y_gain/1 -> FirstOrderFilter8/3  "VTQD_HVBCurrSmooth_gain"
  FirstOrderFilter8/1 -> Switch/1
  [VINP_HVBPwrAvailDchrgValid_flg] -> Switch/2
  Constant2/1 -> Data Type Conversion/1
  Data Type Conversion/1 -> Switch/3
  Max/1 -> Divide/3
  Constant1/1 -> Max/1
  Constant3/1 -> Max/2
  [VINP_B2VPackInsideVol_V] -> Divide/2
  [VINP_B2VAPlsDischgCurr_A] -> Divide/1
  Divide/1 -> [VTQD_HVBPwrAvailDchrg_kW]  "VTQD_HVBPwrAvailDchrg_kW"
  Constant5/1 -> Max1/2
  [VINP_B2VPackInsideVol_V] -> Divide1/2
  Divide1/1 -> [VTQD_HVBattPwrAvailChrg_kW]  "VTQD_HVBattPwrAvailChrg_kW"
  Max1/1 -> Divide1/3
  [VINP_B2VAvaPlsChgCurr_A] -> Divide1/1
  Constant4/1 -> Max1/1
  [VINP_MotorSpd_rpm] -> Abs1/1
  Mux1/1 -> Fcn1/1
  Fcn1/1 -> Saturaton3/1
  Saturaton2/1 -> Mux1/2
  [VTQD_HVBattPwrAvailChrg_kW] -> Mux1/1
  Abs1/1 -> Saturaton2/1
  Saturaton3/1 -> Gain/1
  Gain/1 -> [VTQD_HVBChrgLim_Nm]  "VTQD_HVBChrgLim_Nm"
  [VTQD_HVBChrgLim_Nm] -> Switch1/1
  Constant6/1 -> Data Type Conversion1/1
  Data Type Conversion1/1 -> Switch1/3
  [VINP_B2VAvaPlsChgCurrValid_flg] -> Switch1/2
  [VTQD_TMTqCapMot_Nm] -> VTQD_TMTqCapMot_Nm/1
  [VTQD_TMTqCapGen_Nm] -> VTQD_TMTqCapGen_Nm/1
  Bus Selector1/1 -> [task_time_s]  "<task_time_s>"
  BSCPIn_outputs/1 -> Bus Selector1/1
  BSignalConvert_outputs/1 -> Terminator/1
  Bus Selector1/2 -> [VINP_B2VAvaPlsChgCurr_A]  "<VINP_B2VAvaPlsChgCurr_A>"
  Bus Selector1/3 -> [VINP_MotorSpd_rpm]  "<VINP_MotorSpd_rpm>"
  Bus Selector1/4 -> [VINP_B2VAPlsDischgCurr_A]  "<VINP_B2VAPlsDischgCurr_A>"
  Bus Selector1/5 -> [VINP_B2VPackInsideVol_V]  "<VINP_B2VPackInsideVol_V>"
  Bus Selector1/6 -> [VINP_B2VPackCurr_A]  "<VINP_B2VPackCurr_A>"
  Bus Selector1/7 -> [VINP_HVBPwrAvailDchrgValid_flg]  "<VINP_HVBPwrAvailDchrgValid_flg>"
  Bus Selector1/8 -> [VINP_B2VAvaPlsChgCurrValid_flg]  "<VINP_B2VAvaPlsChgCurrValid_flg>"
  Bus Selector1/9 -> [VINP_MCUTrqLimHi_Nm]  "<VINP_MCUTrqLimHi_Nm>"
  Bus Selector1/10 -> [VINP_MCUTrqLimLo_Nm]  "<VINP_MCUTrqLimLo_Nm>"
  Min/1 -> [VTQD_TMTqCapMot_Nm]  "VTQD_TMTqCapMot_Nm"
  [VINP_MCUTrqLimHi_Nm] -> Min/2
  Switch/1 -> Min/1
  Switch1/1 -> Min1/1
  [VINP_MCUTrqLimLo_Nm] -> Min1/2
  Min1/1 -> [VTQD_TMTqCapGen_Nm]  "VTQD_TMTqCapGen_Nm"

== system tqd/TQD/Input_Convert/Input Signal Convert/Big Mike Combo V2  ==
  task_time_s : Inport
  VACC_ASC2NLvReqFA_enum : Inport  Port=2
  VACC_ASC2NLvReqRA_enum : Inport  Port=3
  VACC_ASC2KneeReqRSide_flg : Inport  Port=4
  VACC_ASC2KneeReqFA_flg : Inport  Port=5
  VACC_ASC2KneeReqRA_flg : Inport  Port=6
  VBCM_FDCBCMFDCloseSVCmd_flg : Inport  Port=7
  VBCM_FDCBCMFDOpenSVCmd_flg : Inport  Port=8
  VINP_TransReqGear_enum : Inport  Port=9
  VINP_ParkBrakeSW_flg : Inport  Port=10
  VINP_BrakePedalPos_pct : Inport  Port=11
  VDHP_ActAPSPosn_pct : Inport  Port=12
  VPMM_SysPowerMode_enum : Inport  Port=13
  VTQD_GearActualPosn_enum : Inport  Port=14
  VTQD_ActFRDoorOPSta_flg : Inport  Port=15
  Combo Key Detection : Subsystem
      settings: RTWSystemCode=Nonreusable function
  Mode Coordination : Subsystem  TreatAsAtomicUnit=on
      settings: RTWSystemCode=Nonreusable function
  Operation Condition : Subsystem
      settings: RTWSystemCode=Nonreusable function
  Signal Status Detection : Subsystem
      settings: RTWSystemCode=Nonreusable function
  VTQD_Function1Off_flg : Outport
  VTQD_Function2Off_flg : Outport  Port=2
  VTQD_Function3Off_flg : Outport  Port=3
  VTQD_Function4Off_flg : Outport  Port=4
  VTQD_Function5Off_flg : Outport  Port=5
  VTQD_ComboKeyEn_flg : Outport  Port=6
  VTQD_ComboKeyPreEn_flg : Outport  Port=7
  VTQD_FunctionOffSta_enum : Outport  Port=8
  wires:
  Signal Status Detection/1(VTQD_ComboKey_enum) -> [VTQD_ComboKey_enum]
  [VTQD_Function1Off_flg] -> VTQD_Function1Off_flg/1
  Operation Condition/1(VTQD_ComboKeyPreEn_flg) -> [VTQD_ComboKeyPreEn_flg]
  VACC_ASC2NLvReqRA_enum/1 -> [VACC_ASC2NLvReqRA_enum]
  [VTQD_ComboKeyEnCMD_flg] -> Operation Condition/3(VTQD_ComboKeyEnCMD_flg)
  Signal Status Detection/4(VTQD_ComboKeyEnter_flg) -> [VTQD_ComboKeyEnter_flg]
  VACC_ASC2NLvReqFA_enum/1 -> [VACC_ASC2NLvReqFA_enum]
  VACC_ASC2KneeReqFA_flg/1 -> [VACC_ASC2KneeReqFA_flg]
  Signal Status Detection/2(VTQD_ComboKeyEnCMD_flg) -> [VTQD_ComboKeyEnCMD_flg]
  Operation Condition/2(VTQD_ComboKeyEn_flg) -> [VTQD_ComboKeyEn_flg]
  VPMM_SysPowerMode_enum/1 -> [VPMM_SysPowerMode_enum]
  VINP_TransReqGear_enum/1 -> [VINP_TransReqGear_enum]
  [VTQD_GearActualPosn_enum] -> Operation Condition/2(VTQD_GearActualPosn_enum)
  Signal Status Detection/3(VTQD_ComboKeyReset_flg) -> [VTQD_ComboKeyReset_flg]
  VTQD_GearActualPosn_enum/1 -> [VTQD_GearActualPosn_enum]
  Signal Status Detection/5(VTQD_ComboKeyOff_flg) -> [VTQD_ComboKeyOff_flg]
  VACC_ASC2KneeReqRSide_flg/1 -> [VACC_ASC2KneeReqRSide_flg]
  VACC_ASC2KneeReqRA_flg/1 -> [VACC_ASC2KneeReqRA_flg]
  task_time_s/1 -> [task_time_s]
  VBCM_FDCBCMFDCloseSVCmd_flg/1 -> [VBCM_FDCBCMFDCloseSVCmd_flg]
  VBCM_FDCBCMFDOpenSVCmd_flg/1 -> [VBCM_FDCBCMFDOpenSVCmd_flg]
  VINP_BrakePedalPos_pct/1 -> [VINP_BrakePedalPos_pct]
  VDHP_ActAPSPosn_pct/1 -> [VDHP_ActAPSPosn_pct]
  [VTQD_ComboKeyPreEn_flg] -> VTQD_ComboKeyPreEn_flg/1
  [VTQD_ComboKeyEn_flg] -> VTQD_ComboKeyEn_flg/1
  [VTQD_ComboKeyEn_flg] -> Signal Status Detection/14(VTQD_ComboKeyEn_flg)
  Combo Key Detection/1(VTQD_Function1Off_flg) -> [VTQD_Function1Off_flg]
  [task_time_s] -> Combo Key Detection/1(task_time_s)
  [VTQD_ComboKeyEn_flg] -> Combo Key Detection/2(VTQD_ComboKeyEn_flg)
  [VTQD_ComboKeyReset_flg] -> Combo Key Detection/3(VTQD_ComboKeyReset_flg)
  [VTQD_ComboKey_enum] -> Combo Key Detection/4(VTQD_ComboKey_enum)
  [VTQD_ComboKeyEnter_flg] -> Combo Key Detection/5(VTQD_ComboKeyEnter_flg)
  [VTQD_ComboKeyOff_flg] -> Combo Key Detection/6(VTQD_ComboKeyOff_flg)
  [VTQD_Function2Off_flg] -> VTQD_Function2Off_flg/1
  Combo Key Detection/2(VTQD_Function2Off_flg) -> [VTQD_Function2Off_flg]
  Combo Key Detection/3(VTQD_Function3Off_flg) -> [VTQD_Function3Off_flg]
  [VTQD_Function3Off_flg] -> VTQD_Function3Off_flg/1
  Combo Key Detection/4(VTQD_Function4Off_flg) -> [VTQD_Function4Off_flg]
  [VTQD_Function4Off_flg] -> VTQD_Function4Off_flg/1
  Combo Key Detection/5(VTQD_Function5Off_flg) -> [VTQD_Function5Off_flg]
  [VTQD_Function5Off_flg] -> VTQD_Function5Off_flg/1
  [VTQD_Function1Off_flg] -> Mode Coordination/1(VTQD_Function1Off_flg)
  [VTQD_Function2Off_flg] -> Mode Coordination/2(VTQD_Function2Off_flg)
  [VTQD_Function3Off_flg] -> Mode Coordination/3(VTQD_Function3Off_flg)
  [VTQD_Function4Off_flg] -> Mode Coordination/4(VTQD_Function4Off_flg)
  [VTQD_Function5Off_flg] -> Mode Coordination/5(VTQD_Function5Off_flg)
  Mode Coordination/1(VTQD_FunctionOffSta_enum) -> [VTQD_FunctionOffSta_enum]
  [VTQD_FunctionOffSta_enum] -> VTQD_FunctionOffSta_enum/1
  [VTQD_ActFRDoorOPSta_flg] -> Operation Condition/5(VTQD_ActFRDoorOPSta_flg)
  VTQD_ActFRDoorOPSta_flg/1 -> [VTQD_ActFRDoorOPSta_flg]
  VINP_ParkBrakeSW_flg/1 -> [VINP_ParkBrakeSW_flg]
  [task_time_s] -> Signal Status Detection/1(task_time_s)
  [VTQD_ComboKeyPreEn_flg] -> Signal Status Detection/9(VTQD_ComboKeyPreEn_flg)
  [VTQD_FunctionOffSta_enum] -> Signal Status Detection/11(VTQD_FunctionOffSta_enum)
  [VTQD_ActFRDoorOPSta_flg] -> Signal Status Detection/15(VTQD_ActFRDoorOPSta_flg)
  [VACC_ASC2NLvReqFA_enum] -> Signal Status Detection/2(VACC_ASC2NLvReqFA_enum)
  [VACC_ASC2NLvReqRA_enum] -> Signal Status Detection/3(VACC_ASC2NLvReqRA_enum)
  [VACC_ASC2KneeReqRSide_flg] -> Signal Status Detection/4(VACC_ASC2KneeReqRSide_flg)
  [VACC_ASC2KneeReqFA_flg] -> Signal Status Detection/5(VACC_ASC2KneeReqFA_flg)
  [VACC_ASC2KneeReqRA_flg] -> Signal Status Detection/6(VACC_ASC2KneeReqRA_flg)
  [VBCM_FDCBCMFDCloseSVCmd_flg] -> Signal Status Detection/7(VBCM_FDCBCMFDCloseSVCmd_flg)
  [VBCM_FDCBCMFDOpenSVCmd_flg] -> Signal Status Detection/8(VBCM_FDCBCMFDOpenSVCmd_flg)
  [VINP_TransReqGear_enum] -> Signal Status Detection/10(VINP_TransReqGear_enum)
  [VDHP_ActAPSPosn_pct] -> Signal Status Detection/12(VDHP_ActAPSPosn_pct)
  [VINP_BrakePedalPos_pct] -> Signal Status Detection/13(VINP_BrakePedalPos_pct)
  [VINP_ParkBrakeSW_flg] -> Operation Condition/4(VINP_ParkBrakeSW_flg)
  [VPMM_SysPowerMode_enum] -> Operation Condition/1(VPMM_SysPowerMode_enum)

== system tqd/TQD/Input_Convert/Input Signal Convert/Engineering Mode Disable Flasher ==
  Task_Time_s : Inport
  ON_s : Inport  Port=2
  OFF_s : Inport  Port=3
  Cycle_cnt : Inport  Port=4
  Wait_s : Inport  Port=5
  VSCP_FlasherEn_flg : Inport  Port=6
  Add : Sum  Inputs=+-
  Chart : Stateflow chart  TreatAsAtomicUnit=on
  Constant4 : Constant  Value=ONE_INT
  Data Type Conversion{,1..3} (4 alike) : DataTypeConversion  OutDataTypeStr=uint8
  Divide : Product  Inputs=*/
  Divide1 : Product  Inputs=*/
  Divide2 : Product  Inputs=*/
  Floor : Rounding
  Floor1 : Rounding
  Floor2 : Rounding
  SigOut : Outport
  wires:
  Floor2/1 -> Data Type Conversion2/1  "WAIT_cnt"
  Floor1/1 -> Data Type Conversion1/1  "OFF_cnt"
  Divide/1 -> Floor/1
  Divide1/1 -> Floor1/1
  Add/1 -> Data Type Conversion3/1  "Cycle_cnt"
  Floor/1 -> Data Type Conversion/1  "ON_cnt"
  Divide2/1 -> Floor2/1
  Constant4/1 -> Add/2
  [Cycle_cnt] -> Add/1  "Cycle_cnt"
  ON_s/1 -> [ON_s]
  OFF_s/1 -> [OFF_s]
  [TaskTime_s] -> Divide/2
  [TaskTime_s] -> Divide2/2
  [Wait_s] -> Divide2/1  "Wait_s"
  [TaskTime_s] -> Divide1/2
  [ON_s] -> Divide/1  "ON_s"
  [OFF_s] -> Divide1/1  "OFF_s"
  Cycle_cnt/1 -> [Cycle_cnt]
  Wait_s/1 -> [Wait_s]
  Chart/1(out) -> SigOut/1
  Task_Time_s/1 -> [TaskTime_s]
  VSCP_FlasherEn_flg/1 -> [VSCP_FlasherEn_flg]
  [VSCP_FlasherEn_flg] -> Chart/5(VSCP_FlasherEn_flg)
  Data Type Conversion/1 -> Chart/1(ON_cnt)
  Data Type Conversion1/1 -> Chart/2(OFF_cnt)
  Data Type Conversion2/1 -> Chart/3(WAIT_cnt)
  Data Type Conversion3/1 -> Chart/4(Cycle_cnt)

== system tqd/TQD/Input_Convert/Input Signal Convert/Engineering Mode Enable Flasher ==
  Task_Time_s : Inport
  ON_s : Inport  Port=2
  OFF_s : Inport  Port=3
  Cycle_cnt : Inport  Port=4
  Wait_s : Inport  Port=5
  VSCP_FlasherEn_flg : Inport  Port=6
  Add : Sum  Inputs=+-
  Chart : Stateflow chart  TreatAsAtomicUnit=on
  Constant4 : Constant  Value=ONE_INT
  Data Type Conversion{,1..3} (4 alike) : DataTypeConversion  OutDataTypeStr=uint8
  Divide : Product  Inputs=*/
  Divide1 : Product  Inputs=*/
  Divide2 : Product  Inputs=*/
  Floor : Rounding
  Floor1 : Rounding
  Floor2 : Rounding
  SigOut : Outport
  wires:
  Floor2/1 -> Data Type Conversion2/1  "WAIT_cnt"
  Floor1/1 -> Data Type Conversion1/1  "OFF_cnt"
  Divide/1 -> Floor/1
  Divide1/1 -> Floor1/1
  Add/1 -> Data Type Conversion3/1  "Cycle_cnt"
  Floor/1 -> Data Type Conversion/1  "ON_cnt"
  Divide2/1 -> Floor2/1
  Constant4/1 -> Add/2
  [Cycle_cnt] -> Add/1  "Cycle_cnt"
  ON_s/1 -> [ON_s]
  OFF_s/1 -> [OFF_s]
  [TaskTime_s] -> Divide/2
  [TaskTime_s] -> Divide2/2
  [Wait_s] -> Divide2/1  "Wait_s"
  [TaskTime_s] -> Divide1/2
  [ON_s] -> Divide/1  "ON_s"
  [OFF_s] -> Divide1/1  "OFF_s"
  Cycle_cnt/1 -> [Cycle_cnt]
  Wait_s/1 -> [Wait_s]
  Chart/1(out) -> SigOut/1
  Task_Time_s/1 -> [TaskTime_s]
  VSCP_FlasherEn_flg/1 -> [VSCP_FlasherEn_flg]
  [VSCP_FlasherEn_flg] -> Chart/5(VSCP_FlasherEn_flg)
  Data Type Conversion/1 -> Chart/1(ON_cnt)
  Data Type Conversion1/1 -> Chart/2(OFF_cnt)
  Data Type Conversion2/1 -> Chart/3(WAIT_cnt)
  Data Type Conversion3/1 -> Chart/4(Cycle_cnt)

== system tqd/TQD/Input_Convert/Input Signal Convert/Flasher ==
  triger : Inport
  FlashTime : Inport  Port=2
  Add : Sum
  Constant1 : Constant  Value=TRUE
  Constant2 : Constant  Value=FALSE
  Constant3 : Constant  Value=FALSE
  Constant4 : Constant  Value=ONE_INT
  Constant5 : Constant  Value=ZERO_INT
  Constant6 : Constant  Value=ONE_INT
  Data Type Conversion : DataTypeConversion  OutDataTypeStr=uint8
  Data Type Conversion1 : DataTypeConversion  OutDataTypeStr=boolean
  Delay : Delay  DelayLength=1  InitialCondition=uint8(0)
      settings: AttributesFormatString=%<InitialCondition>
  Delay1 : Delay  DelayLength=1  InitialCondition=boolean(0)
      settings: AttributesFormatString=%<InitialCondition>
  Relational Operator : RelationalOperator  Operator=>  OutDataTypeStr=boolean  RndMeth=Simplest
  Switch{,1..2,4} (4 alike) : Switch  Criteria=u2 ~= 0
      settings: AttributesFormatString=%<Criteria>
  Switch3 : Switch  Criteria=u2 > Threshold
  Result : Outport
  wires:
  [triger] -> Switch4/2
  [triger] -> Switch3/2
  triger/1 -> [triger]
  Switch4/1 -> Switch1/3
  FlashTime/1 -> Relational Operator/2
  Add/1 -> Switch3/1
  [Result_delay] -> Switch/2
  Delay/1 -> Data Type Conversion/1
  Switch2/1 -> Delay/1
  Constant1/1 -> Switch/3
  Delay1/1 -> Data Type Conversion1/1
  Switch/1 -> Switch1/1
  Constant2/1 -> Switch/1
  Relational Operator/1 -> Switch1/2, Switch2/2
  Switch3/1 -> Switch2/3, Relational Operator/1
  Constant6/1 -> Add/1
  Switch1/1 -> Result/1, Delay1/1
  Constant5/1 -> Switch3/3
  Constant3/1 -> Switch4/3
  Data Type Conversion/1 -> Add/2
  Data Type Conversion1/1 -> Switch4/1, [Result_delay]
  Constant4/1 -> Switch2/1

== system tqd/TQD/Input_Convert/Input Signal Convert/kph to rpm  ==
  SetSpeed_kph : Inport
  Constant : Constant  Value=THOUSAND
  Constant1 : Constant  Value=KTQD_VehSpdGearRatio_ratio
  Constant2 : Constant  Value=SIXTY
  Constant3 : Constant  Value=KTQD_VehSpdTireDiameter_m
  Constant4 : Constant  Value=KTQD_VehSpdTireFactor_Factor
  Constant5 : Constant  Value=KTQD_VehSpdADJFactor_Factor
  Constant57 : Constant  Value=KTQD_VCUMCUDemHiPosVal_rpm
  Constant{6..9} (4 alike) : Constant  Value=EPS  OutDataTypeStr=single
  Divide : Product  Inputs=*////
  Max{,1..3} (4 alike) : MinMax  Function=max  Inputs=2
  Min : MinMax  Inputs=2
  Product : Product  Inputs=3
  MotorSpd_rpm : Outport
  wires:
  Constant/1 -> Product/2
  SetSpeed_kph/1 -> Product/1
  Product/1 -> Divide/1
  Constant1/1 -> Product/3
  Divide/1 -> Min/1
  Min/1 -> MotorSpd_rpm/1
  Constant57/1 -> Min/2
  Max/1 -> Divide/2
  Constant2/1 -> Max/1
  Constant6/1 -> Max/2
  Max1/1 -> Divide/3
  Constant3/1 -> Max1/1
  Constant7/1 -> Max1/2
  Constant8/1 -> Max2/2
  Max2/1 -> Divide/4
  Constant4/1 -> Max2/1
  Constant9/1 -> Max3/2
  Max3/1 -> Divide/5
  Constant5/1 -> Max3/1

== system tqd/TQD/OutpConvert/Buzzer Request/Combo Key Flasher ==
  Task_Time_s : Inport
  ON_s : Inport  Port=2
  OFF_s : Inport  Port=3
  Cycle_cnt : Inport  Port=4
  Wait_s : Inport  Port=5
  VSCP_FlasherEn_flg : Inport  Port=6
  Add : Sum  Inputs=+-
  Chart : Stateflow chart  TreatAsAtomicUnit=on
  Constant4 : Constant  Value=ONE_INT
  Data Type Conversion{,1..3} (4 alike) : DataTypeConversion  OutDataTypeStr=uint8
  Divide : Product  Inputs=*/
  Divide1 : Product  Inputs=*/
  Divide2 : Product  Inputs=*/
  Floor : Rounding
  Floor1 : Rounding
  Floor2 : Rounding
  SigOut : Outport
  wires:
  Floor/1 -> Data Type Conversion/1  "ON_cnt"
  [TaskTime_s] -> Divide2/2
  [Cycle_cnt] -> Add/1  "Cycle_cnt"
  VSCP_FlasherEn_flg/1 -> [VSCP_FlasherEn_flg]
  [VSCP_FlasherEn_flg] -> Chart/5(VSCP_FlasherEn_flg)
  Wait_s/1 -> [Wait_s]
  Task_Time_s/1 -> [TaskTime_s]
  OFF_s/1 -> [OFF_s]
  Cycle_cnt/1 -> [Cycle_cnt]
  [TaskTime_s] -> Divide/2
  [Wait_s] -> Divide2/1  "Wait_s"
  [OFF_s] -> Divide1/1  "OFF_s"
  Constant4/1 -> Add/2
  Data Type Conversion3/1 -> Chart/4(Cycle_cnt)
  ON_s/1 -> [ON_s]
  Divide1/1 -> Floor1/1
  Floor2/1 -> Data Type Conversion2/1  "WAIT_cnt"
  [ON_s] -> Divide/1  "ON_s"
  Data Type Conversion/1 -> Chart/1(ON_cnt)
  Chart/1(out) -> SigOut/1
  Data Type Conversion1/1 -> Chart/2(OFF_cnt)
  Data Type Conversion2/1 -> Chart/3(WAIT_cnt)
  Floor1/1 -> Data Type Conversion1/1  "OFF_cnt"
  Add/1 -> Data Type Conversion3/1  "Cycle_cnt"
  Divide/1 -> Floor/1
  [TaskTime_s] -> Divide1/2
  Divide2/1 -> Floor2/1
